simulink model "SMR_draft2"  (R2024a)
settings: Solver=VariableStepAuto  StartTime=0.0  StopTime=60*30  RelTol=1e-3
undefined symbols (not defined in the file): area_air, cp_air, HC_min, HC_nom, rho_air, vel_air_nom
libraries: fl_lib x32, nesl_utility x20, SimscapeFluids_lib x6, simulink x3, RankineCycle_lib x1
(part 2 of 2)

== system SMR_draft2/Steam Condenser/Sensor air out ==
  Mass & Energy Flow Rate Sensor (MA) : fl_lib/Moist Air/Sensors/Flow Rate Sensor (MA)  mass_flow_measure=true  volumetric_flow_measure=false  volumetric_flow_conditions=foundation.enum.volumetric_flow_conditions.actual  p_std=0.101325 MPa  T_std=20 degC  RH_std=0.65  energy_flow_measure=true  vapor_flow_measure=true  gas_flow_measure=true
      settings: InternalSimscapePortConfiguration="{\"Bottom\":[{\"id\":\"PHI\",\"label\":\"φ\",\"type\":\"output\"}],\"Left\":[{\"id\":\"A\",\"label\":\"A\",\"type\":\"foundation.moist_air.moist_air\"},{\"id\":\"Mw\",\"label\":\"Mw\",\"type\":\"output\"},{\"id\":\"Mg\",\"label\":\"Mg\",\"type\":\"output\"}],\"Right\":[{\"id\":\"B\",\"label\":\"B\",\"type\":\"foundation.moist_air.moist_air\"},{\"id\":\"M\",\"label\":\"M\",\"type\":\"output\"}],\"Top\":[]}"
  PS-Simulink Converter : nesl_utility/PS-Simulink Converter  PhysicalDomain=network_engine_domain  SubClassName=ps_output  LeftPortType=input  RightPortType=output  PseudoPeriodic=off  Frequencies=[]  VectorFormat=1-D array  Unit=kW  AffineConversion=off
  A : PMIOPort  Side=Left
  B : PMIOPort  Port=2  Side=Right
  tag scope: Phi_air_out=global
  wires:
  PS-Simulink Converter/1 -> [Phi_air_out]
  connections:
  Mass & Energy Flow Rate Sensor (MA)/RConn1 -- B/RConn1
  Mass & Energy Flow Rate Sensor (MA)/LConn1 -- A/RConn1
  Mass & Energy Flow Rate Sensor (MA)/RConn3 -- PS-Simulink Converter/LConn1

== system SMR_draft2/Steam Condenser/Sensor condensate ==
  PS-Simulink Converter : nesl_utility/PS-Simulink Converter  PhysicalDomain=network_engine_domain  SubClassName=ps_output  LeftPortType=input  RightPortType=output  PseudoPeriodic=off  Frequencies=[]  VectorFormat=1-D array  Unit=g/s  AffineConversion=off
  A : PMIOPort  Side=Left
  tag scope: mdot_water=global
  wires:
  PS-Simulink Converter/1 -> [mdot_water]
  connections:
  A/RConn1 -- PS-Simulink Converter/LConn1

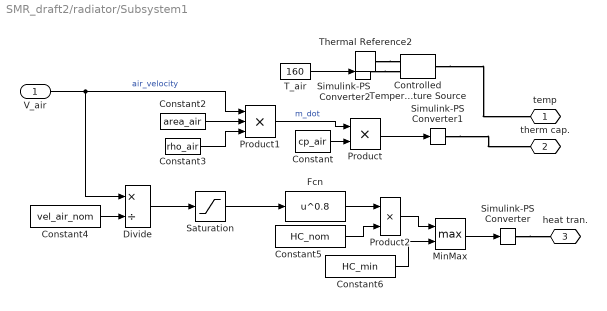
== system SMR_draft2/radiator/Subsystem1 ==
  V_air : Inport
  Constant : Constant  Value=cp_air
  Constant2 : Constant  Value=area_air
  Constant3 : Constant  Value=rho_air
  Constant4 : Constant  Value=vel_air_nom
  Constant5 : Constant  Value=HC_nom
  Constant6 : Constant  Value=HC_min
  Controlled Temperature Source : fl_lib/Thermal/Thermal Sources/Controlled Temperature Source
  Divide : Product  Inputs=*/
  Fcn : Fcn  Expr=u^0.8
  MinMax : MinMax  Function=max  Inputs=2
  Product : Product
  Product1 : Product  Inputs=3
  Product2 : Product
  Saturation : Saturate  UpperLimit=inf  LowerLimit=0
  Simulink-PS Converter : nesl_utility/Simulink-PS Converter  PhysicalDomain=network_engine_domain  SubClassName=ps_input  LeftPortType=input  RightPortType=output  PseudoPeriodic=off  Frequencies=[]  NoiseDistribution=none  NoiseParameters=[]  Unit=1  AffineConversion=off  FilteringAndDerivatives=provide  SimscapeFilterOrder=1  InputFilterTimeConstant=0.001  UdotUserProvided=0
  Simulink-PS Converter1 : nesl_utility/Simulink-PS Converter  PhysicalDomain=network_engine_domain  SubClassName=ps_input  LeftPortType=input  RightPortType=output  PseudoPeriodic=off  Frequencies=[]  NoiseDistribution=none  NoiseParameters=[]  Unit=1  AffineConversion=off  FilteringAndDerivatives=provide  SimscapeFilterOrder=1  InputFilterTimeConstant=0.001  UdotUserProvided=0
  Simulink-PS Converter2 : nesl_utility/Simulink-PS Converter  PhysicalDomain=network_engine_domain  SubClassName=ps_input  LeftPortType=input  RightPortType=output  PseudoPeriodic=off  Frequencies=[]  NoiseDistribution=none  NoiseParameters=[]  Unit=1  AffineConversion=off  FilteringAndDerivatives=provide  SimscapeFilterOrder=1  InputFilterTimeConstant=0.001  UdotUserProvided=0
  T_air : Constant  Value=160
  Thermal Reference2 : fl_lib/Thermal/Thermal Elements/Thermal Reference
  temp : PMIOPort  Side=Left
  therm cap. : PMIOPort  Port=2  Side=Left
  heat tran. : PMIOPort  Port=3  Side=Left
  wires:
  MinMax/1 -> Simulink-PS Converter/1
  Constant/1 -> Product/2
  T_air/1 -> Simulink-PS Converter2/1
  Product/1 -> Simulink-PS Converter1/1
  Product1/1 -> Product/1  "m_dot"
  Constant2/1 -> Product1/2
  Constant3/1 -> Product1/3
  V_air/1 -> Divide/1, Product1/1  "air_velocity"
  Saturation/1 -> Fcn/1
  Divide/1 -> Saturation/1
  Constant6/1 -> MinMax/2
  Product2/1 -> MinMax/1
  Fcn/1 -> Product2/1
  Constant5/1 -> Product2/2
  Constant4/1 -> Divide/2
  connections:
  Thermal Reference2/LConn1 -- Controlled Temperature Source/RConn2
  Controlled Temperature Source/LConn1 -- temp/RConn1
  Simulink-PS Converter2/RConn1 -- Controlled Temperature Source/RConn1
  Simulink-PS Converter1/RConn1 -- therm cap./RConn1
  Simulink-PS Converter/RConn1 -- heat tran./RConn1

== system SMR_draft2/radiator/fan1 ==
  Constant : Constant  Value=250
  Constant1 : Constant  Value=290
  Fan control : Subsystem  mask(2-Level Fan Controller){T_level1=[97 94], T_level2=[105 102]}
      mask prompts: T_level1 "Level 1 temperature"; T_level2 "Level 2 temperature"
      mask help: The primary and secondary fan control temperature ranges are defined by Level 1 temperature vector and Level 2 temperature vector, respectively.
  Fan unit : Subsystem
  V_air : Outport
  wires:
  Fan control/1(U_fan) -> Fan unit/2(U_fan)
  Fan unit/1(V_air) -> V_air/1
  Constant/1 -> Fan control/1(V), Fan unit/1(Veh_speed)
  Constant1/1 -> Fan control/2(T)

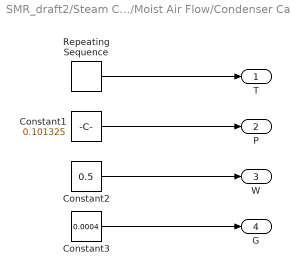
== system SMR_draft2/Steam Condenser/Moist Air Flow/Condenser Case ==
  Constant1 : Constant  Value=0.101325
  Constant2 : Constant  Value=0.5
  Constant3 : Constant  Value=0.0004
  Repeating Sequence : simulink/Sources/Repeating Sequence  rep_seq_t=[0 2000 2500 10000 10500 20000 25000]  rep_seq_y=[25 25 20 20 15 15 25]
  T : Outport
  P : Outport  Port=2
  W : Outport  Port=3
  G : Outport  Port=4
  wires:
  Constant1/1 -> P/1
  Constant2/1 -> W/1
  Repeating Sequence/1 -> T/1
  Constant3/1 -> G/1

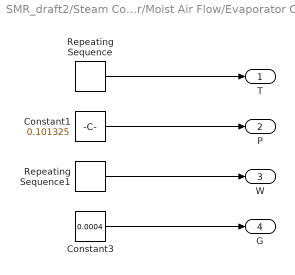
== system SMR_draft2/Steam Condenser/Moist Air Flow/Evaporator Case ==
  Constant1 : Constant  Value=0.101325
  Constant3 : Constant  Value=0.0004
  Repeating Sequence : simulink/Sources/Repeating Sequence  rep_seq_t=[0 200 300 600 700 800 900]  rep_seq_y=[25 25 35 35 30 30 25]
  Repeating Sequence1 : simulink/Sources/Repeating Sequence  rep_seq_t=[0 400 500 800 900]  rep_seq_y=[0 0 0.5 0.5 0]
  T : Outport
  P : Outport  Port=2
  W : Outport  Port=3
  G : Outport  Port=4
  wires:
  Repeating Sequence1/1 -> W/1
  Repeating Sequence/1 -> T/1
  Constant3/1 -> G/1
  Constant1/1 -> P/1

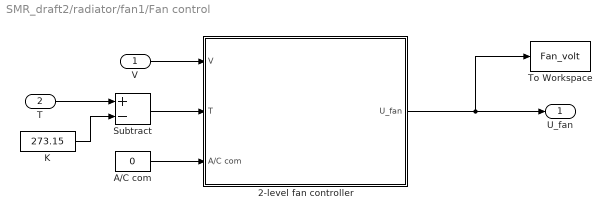
== system SMR_draft2/radiator/fan1/Fan control ==
  V : Inport
  T : Inport  Port=2
  2-level fan controller : Subsystem
  A/C com : Constant  Value=0
  K : Constant  Value=273.15
  Subtract : Sum  Inputs=+-
  To Workspace : ToWorkspace  VariableName=Fan_volt  SampleTime=-1
  U_fan : Outport  VectorParamsAs1DForOutWhenUnconnected=off
  wires:
  K/1 -> Subtract/2
  T/1 -> Subtract/1
  A/C com/1 -> 2-level fan controller/3(A/C com)
  Subtract/1 -> 2-level fan controller/2(T)
  V/1 -> 2-level fan controller/1(V)
  2-level fan controller/1(U_fan) -> To Workspace/1, U_fan/1

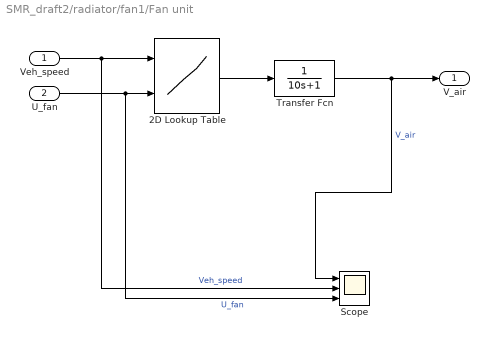
== system SMR_draft2/radiator/fan1/Fan unit ==
  Veh_speed : Inport
  U_fan : Inport  Port=2
  2D Lookup Table : Lookup_n-D  LookupTableObject=''  BreakpointsForDimension1=[0,40,90,110,150,180,198]  BreakpointsForDimension2=[0 14.4]  Table=[0,0.8,2.2,2.7,3.6,4.1,4.6; 1.5,2.3,3.2,3.5,4.3,4.8,5.1]'  InternalRulePriority=Speed  RndMeth=Simplest
      settings: InputPortMap=u0,u1
  Scope : Scope  NumInputPorts=3
  Transfer Fcn : TransferFcn  Denominator=[10 1]
  V_air : Outport  VectorParamsAs1DForOutWhenUnconnected=off
  wires:
  Veh_speed/1 -> Scope/2, 2D Lookup Table/1  "Veh_speed"
  2D Lookup Table/1 -> Transfer Fcn/1
  U_fan/1 -> Scope/3, 2D Lookup Table/2  "U_fan"
  Transfer Fcn/1 -> Scope/1, V_air/1  "V_air"

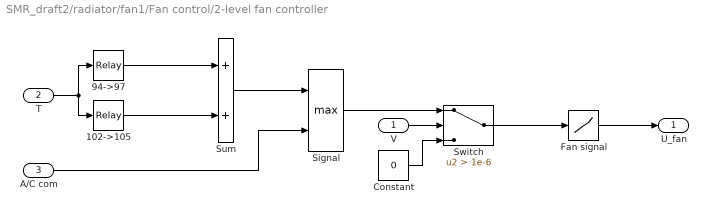
== system SMR_draft2/radiator/fan1/Fan control/2-level fan controller ==
  V : Inport
  T : Inport  Port=2
  A/C com : Inport  Port=3
  102->105 : Relay  OnSwitchValue=T_level2(1)  OffSwitchValue=T_level2(2)
  94->97 : Relay  OnSwitchValue=T_level1(1)  OffSwitchValue=T_level1(2)
  Constant : Constant  Value=0
  Fan signal : Lookup  InputValues=[0, 1, 2]  Table=[0, 5, 14.4]
  Signal : MinMax  Function=max  Inputs=2  InputSameDT=on  SaturateOnIntegerOverflow=on
  Sum : Sum  Inputs=2  InputSameDT=on  SaturateOnIntegerOverflow=on  OutDataTypeStr=Inherit: Same as first input
  Switch : Switch  Criteria=u2 > Threshold  Threshold=1e-6  ZeroCross=off  SaturateOnIntegerOverflow=off  InputSameDT=off
  U_fan : Outport  VectorParamsAs1DForOutWhenUnconnected=off
  wires:
  Fan signal/1 -> U_fan/1
  T/1 -> 102->105/1, 94->97/1
  102->105/1 -> Sum/2
  94->97/1 -> Sum/1
  Sum/1 -> Signal/1
  Signal/1 -> Switch/1
  A/C com/1 -> Signal/2
  V/1 -> Switch/2
  Constant/1 -> Switch/3
  Switch/1 -> Fan signal/1
